simulink model "mod_stream"  (R2023b)
settings: Solver=ode5  StartTime=0.0  StopTime=1  RelTol=1e-3
undefined symbols (not defined in the file or in its folder): Serial_Port, Standard_Devices
libraries: sldrtlib x3
settings Model: Creator=farfar  LastModifiedBy=farfar
settings DataIOCC: ReturnWorkspaceOutputs=off
settings HardwareCC: ProdBitPerLong=64  ProdHWDeviceType=Intel->x86-64 (Linux 64)
settings RTWCC: Description=Simulink Desktop Real-Time  SystemTargetFile=sldrt.tlc  TemplateMakefile=sldrt.tmf  RTWCompilerOptimization=on
settings CodeAppCC: MaxIdLength=95
settings SimulinkDesktopRealTimeCC: TargetLibSuffix=_sldrt.a  TargetPreCompLibLocation=C:\Program Files\MATLAB\R2023b\toolbox\sldrt\lib\win64

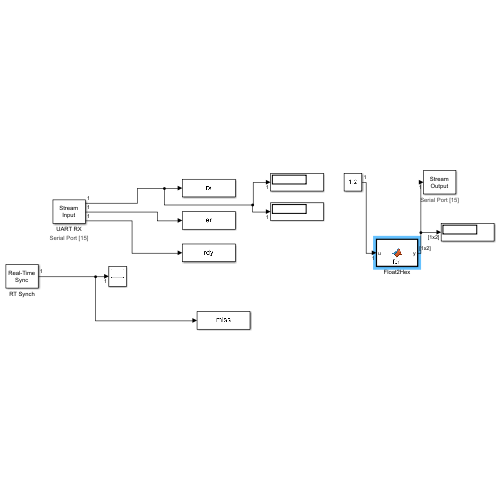
[thumbnail: Simulink's stored preview of the top-level diagram]
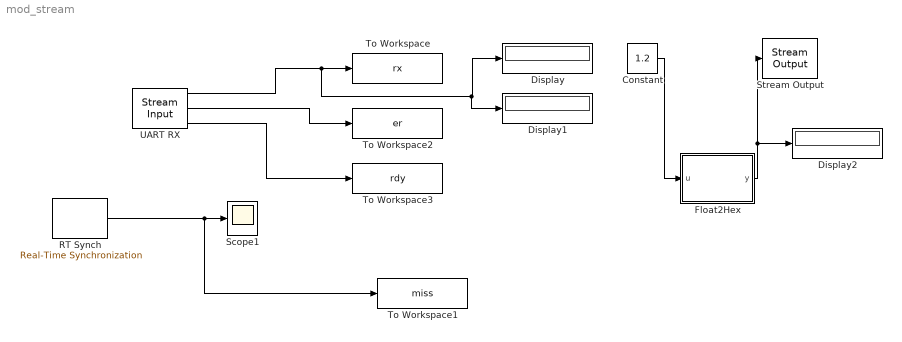
== system mod_stream ==
  Constant : Constant  Value=1.2
  Display : Display
      settings: Format=hex (Stored Integer)
  Display1 : Display
      settings: Format=decimal (Stored Integer)
  Display2 : Display
      settings: Format=hex (Stored Integer)
  Float2Hex : MATLAB Function  TreatAsAtomicUnit=on
  RT Synch : sldrtlib/Real-Time Synchronization  SampleTime=0.004  MaxMissedTicks=10000  ShowMissedTicks=on  YieldWhenWaiting=off
  Scope1 : Scope
  Stream Output : sldrtlib/Stream Output  SampleTime=0.004  MaxMissedTicks=100  ShowMissedTicks=off  YieldWhenWaiting=off  DrvName=Standard_Devices/Serial_Port  DrvAddress=15  DrvOptions=[115200 8 0 0 0 0 0 0]  PortSizes=1  FormatString='%08x\n'  ShowReady=off  ShowError=off  InitialValue=[]  FinalValue=[]
      settings: AttributesFormatString=Serial Port [15]
  To Workspace : ToWorkspace  VariableName=rx  SaveFormat=Structure With Time  SampleTime=-1
  To Workspace1 : ToWorkspace  VariableName=miss  SaveFormat=Structure With Time  SampleTime=-1
  To Workspace2 : ToWorkspace  VariableName=er  SaveFormat=Structure With Time  SampleTime=-1
  To Workspace3 : ToWorkspace  VariableName=rdy  SaveFormat=Structure With Time  SampleTime=-1
  UART RX : sldrtlib/Stream Input  SampleTime=0.004  MaxMissedTicks=10000  ShowMissedTicks=off  YieldWhenWaiting=off  DrvName=Standard_Devices/Serial_Port  DrvAddress=15  DrvOptions=[115200 8 0 0 0 0 0 0]  DataTypes={'uint32'}  FormatString='%x'  Terminator={'\n'}  ShowReady=on  ShowError=on
      settings: AttributesFormatString=Serial Port [15]
  wires:
  UART RX/1 -> Display1/1, Display/1, To Workspace/1
  RT Synch/1 -> To Workspace1/1, Scope1/1
  UART RX/2 -> To Workspace2/1
  UART RX/3 -> To Workspace3/1
  Constant/1 -> Float2Hex/1(u)
  Float2Hex/1(y) -> Stream Output/1, Display2/1

== matlab function mod_stream/Float2Hex ==
  data: u input; y output
function y = fcn(u)
    s = single(u);
    y = typecast(s,'uint32');
